simulink model "Project_Model_simulink_versionSignalBuilder_7_7_2023"  (R2021a)
settings: Solver=FixedStepDiscrete  StartTime=0.0  StopTime=10  FixedStep=0.2  RelTol=1e-3
values from neighbouring files (symbols this model uses):
  Deg_of_Main_Inj = Simulink.Parameter    [Project_Simulink_Parameter_File.m]
  Deg_of_Pre_Inj = Simulink.Parameter    [Project_Simulink_Parameter_File.m]
  Disable = Simulink.Parameter    [Project_Simulink_Parameter_File.m]
  HPP = Simulink.Parameter    [Project_Simulink_Parameter_File.m]
  Increase_percent_Throttle = Simulink.Parameter    [Project_Simulink_Parameter_File.m]
  LPP = Simulink.Parameter    [Project_Simulink_Parameter_File.m]
  Main_Inj_trg_angle_inj1 = Simulink.Parameter    [Project_Simulink_Parameter_File.m]
  Main_Inj_trg_angle_inj2 = Simulink.Parameter    [Project_Simulink_Parameter_File.m]
  Main_Inj_trg_angle_inj3 = Simulink.Parameter    [Project_Simulink_Parameter_File.m]
  Main_Inj_trg_angle_inj4 = Simulink.Parameter    [Project_Simulink_Parameter_File.m]
  Max_RPM = Simulink.Parameter    [Project_Simulink_Parameter_File.m]
  Max_Throttle_Deg = Simulink.Parameter    [Project_Simulink_Parameter_File.m]
  Min_RPM = Simulink.Parameter    [Project_Simulink_Parameter_File.m]
  One_Deg_of_CamRot = Simulink.Parameter    [Project_Simulink_Parameter_File.m]
  Pre_Inj_trg_angle_inj1 = Simulink.Parameter    [Project_Simulink_Parameter_File.m]
  Pre_Inj_trg_angle_inj2 = Simulink.Parameter    [Project_Simulink_Parameter_File.m]
  Pre_Inj_trg_angle_inj3 = Simulink.Parameter    [Project_Simulink_Parameter_File.m]
  Pre_Inj_trg_angle_inj4 = Simulink.Parameter    [Project_Simulink_Parameter_File.m]
  Req_Throttle = Simulink.Parameter    [Project_Simulink_Parameter_File.m]
  RPM_to_CamRPS = Simulink.Parameter    [Project_Simulink_Parameter_File.m]
  RPS_to_timeFactor = Simulink.Parameter    [Project_Simulink_Parameter_File.m]
undefined symbols (not defined in the file or in its folder): sigbuilder_block
(part 2 of 2)

== system Project_Model_simulink_versionSignalBuilder_7_7_2023/CRDI_Integrated_Fuel_Injection_system/Injector_Subsystem/Injector3/Injector_3Subsystem/Pre_injection ==
  Crank_angle : Inport  OutDataTypeStr=single
  Total_ontime_preinjection : Inport  Port=2  OutDataTypeStr=single
  Time_For_1_Degree : Inport  Port=3  OutDataTypeStr=single
  Add : Sum  AccumDataTypeStr=single
      settings: AttributesFormatString=AccumDataTypeStr=%<AccumDataTypeStr>
  Divide : Product  Inputs=*/  OutDataTypeStr=single
  Logical Operator : Logic  AllPortsSameDT=off  OutDataTypeStr=boolean
  Pre_Inj_trg_angle_inj1 : Constant  Value=Pre_Inj_trg_angle_inj3
  Pre_Inj_trg_angle_inj2 : Constant  Value=Pre_Inj_trg_angle_inj3
  Relational Operator : RelationalOperator  OutDataTypeStr=boolean  RndMeth=Simplest
  Relational Operator1 : RelationalOperator  Operator=<=  OutDataTypeStr=boolean  RndMeth=Simplest
  pre_inj_on_off_signal : Outport  VectorParamsAs1DForOutWhenUnconnected=off
  wires:
  Divide/1 -> Add/2
  Relational Operator1/1 -> Logical Operator/2
  Pre_Inj_trg_angle_inj1/1 -> Relational Operator/2  "<Trigger_angle>"
  Total_ontime_preinjection/1 -> Divide/1
  Add/1 -> Relational Operator1/2  "Total_On_Degree"
  Pre_Inj_trg_angle_inj2/1 -> Add/1  "<Trigger_angle>"
  Time_For_1_Degree/1 -> Divide/2
  Relational Operator/1 -> Logical Operator/1
  Crank_angle/1 -> Relational Operator1/1, Relational Operator/1
  Logical Operator/1 -> pre_inj_on_off_signal/1  "pre_inj_on_off_signal"

== system Project_Model_simulink_versionSignalBuilder_7_7_2023/CRDI_Integrated_Fuel_Injection_system/Injector_Subsystem/Injector3/Injector_3Subsystem/Subsystem ==
  note: Subsystem
      | Description: Integrates Pre, Main, Post Injection to single output
      | Input: On time for pre Injection, On time for main Injection, On time for post Injection, Pre Pulse, Main Pulse, Post Pulse
      | Output: On time for Injection
  On_Time_Pre_Injection : Inport
  Pre_Pulse : Inport  Port=2
  On_Time_Main_Injection : Inport  Port=3
  Main_Pulse : Inport  Port=4
  Constant : Constant  Value=Disable
  Switch1 : Switch  Criteria=u2 ~= 0
  Switch2 : Switch  Criteria=u2 ~= 0
  Enable_Disable : Outport  VectorParamsAs1DForOutWhenUnconnected=off
  wires:
  Main_Pulse/1 -> Switch2/2
  On_Time_Main_Injection/1 -> Switch2/1
  Pre_Pulse/1 -> Switch1/2
  On_Time_Pre_Injection/1 -> Switch1/1
  Switch1/1 -> Enable_Disable/1  "On_Time_Injection"
  Constant/1 -> Switch2/3  "constant"
  Switch2/1 -> Switch1/3

== system Project_Model_simulink_versionSignalBuilder_7_7_2023/CRDI_Integrated_Fuel_Injection_system/Injector_Subsystem/Injector4/Injector_4Subsystem/If Action Subsystem ==
  In1 : Inport  OutDataTypeStr=single
  Action Port : ActionPort
  Out1 : Outport  OutDataTypeStr=single
  wires:
  In1/1 -> Out1/1

== system Project_Model_simulink_versionSignalBuilder_7_7_2023/CRDI_Integrated_Fuel_Injection_system/Injector_Subsystem/Injector4/Injector_4Subsystem/If Action Subsystem1 ==
  In1 : Inport  OutDataTypeStr=single
  Action Port : ActionPort
  Out1 : Outport  OutDataTypeStr=single
  wires:
  In1/1 -> Out1/1

== system Project_Model_simulink_versionSignalBuilder_7_7_2023/CRDI_Integrated_Fuel_Injection_system/Injector_Subsystem/Injector4/Injector_4Subsystem/Main_injection ==
  Crank_angle : Inport  OutDataTypeStr=single
  Total_ontime_maininjection : Inport  Port=2  OutDataTypeStr=single
  Time_for_1_Degree : Inport  Port=3  OutDataTypeStr=single
  Add : Sum  AccumDataTypeStr=single
      settings: AttributesFormatString=AccumDataTypeStr=%<AccumDataTypeStr>
  Divide : Product  Inputs=*/  OutDataTypeStr=single
  Logical Operator : Logic  AllPortsSameDT=off  OutDataTypeStr=boolean
  Main_Inj_trg_angle_inj1 : Constant  Value=Main_Inj_trg_angle_inj4
  Main_Inj_trg_angle_inj2 : Constant  Value=Main_Inj_trg_angle_inj4
  Relational Operator : RelationalOperator  OutDataTypeStr=boolean  RndMeth=Simplest
  Relational Operator1 : RelationalOperator  Operator=<=  OutDataTypeStr=boolean  RndMeth=Simplest
  main_inj_on_off_signal : Outport  VectorParamsAs1DForOutWhenUnconnected=off
  wires:
  Logical Operator/1 -> main_inj_on_off_signal/1  "main_inj_on_off_signal"
  Time_for_1_Degree/1 -> Divide/2
  Relational Operator/1 -> Logical Operator/1
  Main_Inj_trg_angle_inj2/1 -> Add/1
  Add/1 -> Relational Operator1/2  "Total_On_Degree"
  Crank_angle/1 -> Relational Operator1/1, Relational Operator/1
  Main_Inj_trg_angle_inj1/1 -> Relational Operator/2
  Relational Operator1/1 -> Logical Operator/2
  Total_ontime_maininjection/1 -> Divide/1
  Divide/1 -> Add/2

== system Project_Model_simulink_versionSignalBuilder_7_7_2023/CRDI_Integrated_Fuel_Injection_system/Injector_Subsystem/Injector4/Injector_4Subsystem/Pre_injection ==
  Crank_angle : Inport  OutDataTypeStr=single
  Total_ontime_preinjection : Inport  Port=2  OutDataTypeStr=single
  Time_For_1_Degree : Inport  Port=3  OutDataTypeStr=single
  Add : Sum  AccumDataTypeStr=single
      settings: AttributesFormatString=AccumDataTypeStr=%<AccumDataTypeStr>
  Divide : Product  Inputs=*/  OutDataTypeStr=single
  Logical Operator : Logic  AllPortsSameDT=off  OutDataTypeStr=boolean
  Pre_Inj_trg_angle_inj1 : Constant  Value=Pre_Inj_trg_angle_inj4
  Pre_Inj_trg_angle_inj2 : Constant  Value=Pre_Inj_trg_angle_inj4
  Relational Operator : RelationalOperator  OutDataTypeStr=boolean  RndMeth=Simplest
  Relational Operator1 : RelationalOperator  Operator=<=  OutDataTypeStr=boolean  RndMeth=Simplest
  pre_inj_on_off_signal : Outport  VectorParamsAs1DForOutWhenUnconnected=off
  wires:
  Divide/1 -> Add/2
  Relational Operator1/1 -> Logical Operator/2
  Pre_Inj_trg_angle_inj1/1 -> Relational Operator/2  "<Trigger_angle>"
  Total_ontime_preinjection/1 -> Divide/1
  Add/1 -> Relational Operator1/2  "Total_On_Degree"
  Pre_Inj_trg_angle_inj2/1 -> Add/1  "<Trigger_angle>"
  Time_For_1_Degree/1 -> Divide/2
  Relational Operator/1 -> Logical Operator/1
  Crank_angle/1 -> Relational Operator1/1, Relational Operator/1
  Logical Operator/1 -> pre_inj_on_off_signal/1  "pre_inj_on_off_signal"

== system Project_Model_simulink_versionSignalBuilder_7_7_2023/CRDI_Integrated_Fuel_Injection_system/Injector_Subsystem/Injector4/Injector_4Subsystem/Subsystem ==
  note: Subsystem
      | Description: Integrates Pre, Main, Post Injection to single output
      | Input: On time for pre Injection, On time for main Injection, On time for post Injection, Pre Pulse, Main Pulse, Post Pulse
      | Output: On time for Injection
  On_Time_Pre_Injection : Inport
  Pre_Pulse : Inport  Port=2
  On_Time_Main_Injection : Inport  Port=3
  Main_Pulse : Inport  Port=4
  Constant : Constant  Value=Disable
  Switch1 : Switch  Criteria=u2 ~= 0
  Switch2 : Switch  Criteria=u2 ~= 0
  Enable_Disable : Outport  VectorParamsAs1DForOutWhenUnconnected=off
  wires:
  Main_Pulse/1 -> Switch2/2
  On_Time_Main_Injection/1 -> Switch2/1
  Pre_Pulse/1 -> Switch1/2
  On_Time_Pre_Injection/1 -> Switch1/1
  Switch1/1 -> Enable_Disable/1  "On_Time_Injection"
  Constant/1 -> Switch2/3  "constant"
  Switch2/1 -> Switch1/3

== matlab function Project_Model_simulink_versionSignalBuilder_7_7_2023/CRDI_Integrated_Fuel_Injection_system/Sensors_Subsystem/Oxygen sensor/MATLAB Function ==
  data: u input; out output
function out = fcn(u)
%#codegen

if (u>0.65)
y = 0.95;
elseif (u<=0.65 && u>=0.25)
    y = 1;
else
    y=1.05;
end

out=y;
